simulink model "Target_Control_System"  (R2021b)
settings: Solver=FixedStepDiscrete  StartTime=0.0  StopTime=5  RelTol=1e-3
PreLoadFcn:
  | RTWConfigurationCB('preloadfcn', bdroot);
PostLoadFcn:
  | load('configuration/data_struct.mat');
  | load('configuration/fluxMaps_propMotor.mat');
  | load('configuration/parameterInit_PROP.mat');
  | load('configuration/parameterInit_PUMP.mat');
  | load('configuration/parameterInit_PITCH.mat');
  | load('configuration/parameterInit_TILT.mat');
  | %load('configuration/base_workspace_signal_definition.mat');
  | %load('resolvedatastores_to_baseworkspace_for_faster_simulation.mat');
model workspace (MAT data in the model file):
  SIMULATION_OPTIONS : Simulink.Parameter (value not decoded)
  TARGET_CODE_GEN : Simulink.Parameter (value not decoded)
  TCS_SAMPLE_FREQ_HZ : Simulink.Parameter (value not decoded)
symbols that are objects in the model workspace (value not decoded): TARGET_CODE_GEN, TCS_SAMPLE_FREQ_HZ
undefined symbols (not defined in the file): A_DQ_REF_LPF_INIT__PITCH, A_DQ_REF_LPF_INIT__PROP, A_DQ_REF_LPF_INIT__PUMP, A_DQ_REF_LPF_INIT__TILT, A_OBSERVER_CONFIDENCE_INIT__PITCH, A_OBSERVER_CONFIDENCE_INIT__PROP, A_OBSERVER_CONFIDENCE_INIT__PUMP, A_OBSERVER_CONFIDENCE_INIT__TILT, ACTUATOR_MAX_ANGLE_TRIP__PITCH, ACTUATOR_MIN_ANGLE_TRIP__PITCH, ACTUATOR_POS_SENSOR_INV_DIRECTION__PITCH, ACTUATOR_POS_SENSOR_INV_DIRECTION__TILT, ACTUATOR_POS_SENSOR_OFFSET__PITCH, ACTUATOR_POS_SENSOR_OFFSET__TILT, ADC_scaler1_baseaddr_TILT, ADC_SCALER_FLOAT_TO_FIXPOINT_EXPANSION, ANGLE_ELEC_FROM_SENSOR_OFFSET_INIT__PITCH, ANGLE_ELEC_FROM_SENSOR_OFFSET_INIT__PROP, ANGLE_ELEC_FROM_SENSOR_OFFSET_INIT__PUMP, ANGLE_ELEC_FROM_SENSOR_OFFSET_INIT__TILT, AUTO_CLEAR_FAULTS_ENABLED__PITCH, AUTO_CLEAR_FAULTS_ENABLED__PROP, AUTO_CLEAR_FAULTS_ENABLED__PUMP, AUTO_CLEAR_FAULTS_ENABLED__TILT, AUTO_CLEAR_FAULTS_WAIT_TICKS__PITCH, AUTO_CLEAR_FAULTS_WAIT_TICKS__PROP, AUTO_CLEAR_FAULTS_WAIT_TICKS__PUMP, AUTO_CLEAR_FAULTS_WAIT_TICKS__TILT, AUTO_I_ZERO_IDLE_TICKS__PITCH, AUTO_I_ZERO_IDLE_TICKS__PROP, AUTO_I_ZERO_IDLE_TICKS__PUMP, AUTO_I_ZERO_IDLE_TICKS__TILT, AUTO_I_ZERO_OFFSET_IDC_THRESHOLD__PITCH, AUTO_I_ZERO_OFFSET_IDC_THRESHOLD__PROP, AUTO_I_ZERO_OFFSET_IDC_THRESHOLD__PUMP, AUTO_I_ZERO_OFFSET_IDC_THRESHOLD__TILT, AUTO_I_ZERO_OFFSET_IPH_THRESHOLD__PITCH, AUTO_I_ZERO_OFFSET_IPH_THRESHOLD__PROP, AUTO_I_ZERO_OFFSET_IPH_THRESHOLD__PUMP, AUTO_I_ZERO_OFFSET_IPH_THRESHOLD__TILT, AUTO_SENSORLESS_SWITCHOVER_DISABLE_OMEGA, AUTO_SENSORLESS_SWITCHOVER_ENABLE_OMEGA, AUTO_SENSORLESS_SWITCHOVER_MIN_CONFIDENCE, AUXILIARY_PROTECTION_UNIT_BASEADDR__TILT, blanking_max_error_omega_INIT_PITCH, blanking_max_error_omega_INIT_TILT, blanking_max_error_position_INIT_PITCH, blanking_max_error_position_INIT_TILT, BRUTE_START_I_Q_REF_RAMP_SPEED__PITCH, BRUTE_START_I_Q_REF_RAMP_SPEED__PROP, BRUTE_START_I_Q_REF_RAMP_SPEED__PUMP, BRUTE_START_I_Q_REF_RAMP_SPEED__TILT, CONTROL_LOOP_DT_INIT__PITCH, CONTROL_LOOP_DT_INIT__PROP, CONTROL_LOOP_DT_INIT__PUMP, CONTROL_LOOP_DT_INIT__TILT, CORRECTION_FILTER_SCALE__PITCH, CORRECTION_FILTER_SCALE__PROP, CORRECTION_FILTER_SCALE__PUMP, CORRECTION_FILTER_SCALE__TILT ... (+458)
libraries: simulink x178, Reusables_Lib x24
(part 42 of 47)

== system Target_Control_System/Target_Control_System/MainLoop/tiltMotor_mainLoop/mainTask_tilt/motorTaskMainFastStep(&oTilt)/Mechanical System - Tilt/processSensors(&oPitch)/Input (motor) side sensor/PosSensorProcess_altImplementations/If Action Subsystem1 ==
  Action Port : ActionPort
  Add6 : Sum
  Constant10 : Constant  Value=-1.5*pi
  Constant11 : Constant  Value=2.0*pi
  Constant9 : Constant  Value=2.0*pi
  Data Store Read20 : DataStoreRead  DataStoreName=oTilt  DataStoreElements=oTilt.oMot_.oState_.oPosSensor_.fAngleElecFromSensor_  IndexOptions=Index vector (dialog)  Indices=1  OutputSizes=1
  Data Store Read21 : DataStoreRead  DataStoreName=oTilt  DataStoreElements=oTilt.oMot_.oState_.oPosSensor_.fAngleElecFromSensorPrevious_  IndexOptions=Index vector (dialog)  Indices=1  OutputSizes=1
  Data Store Read22 : DataStoreRead  DataStoreName=oTilt  DataStoreElements=oTilt.oMot_.oParam_.fIntControlLoopDt_  IndexOptions=Index vector (dialog)  Indices=1  OutputSizes=1
  Data Store Read23 : DataStoreRead  DataStoreName=oTilt  DataStoreElements=oTilt.oMot_.oState_.oPosSensor_.oInputSensorSpeedFilter_.afConstantsA_.h0  IndexOptions=Index vector (dialog)  Indices=1  OutputSizes=1
  Data Store Read24 : DataStoreRead  DataStoreName=oTilt  DataStoreElements=oTilt.oMot_.oState_.oPosSensor_.oInputSensorSpeedFilter_.afConstantsA_.h1  IndexOptions=Index vector (dialog)  Indices=1  OutputSizes=1
  Data Store Read25 : DataStoreRead  DataStoreName=oTilt  DataStoreElements=oTilt.oMot_.oState_.oPosSensor_.oInputSensorSpeedFilter_.afConstantsA_.h2  IndexOptions=Index vector (dialog)  Indices=1  OutputSizes=1
  Data Store Read26 : DataStoreRead  DataStoreName=oTilt  DataStoreElements=oTilt.oMot_.oState_.oPosSensor_.oInputSensorSpeedFilter_.afConstantsB_.h0  IndexOptions=Index vector (dialog)  Indices=1  OutputSizes=1
  Data Store Read27 : DataStoreRead  DataStoreName=oTilt  DataStoreElements=oTilt.oMot_.oState_.oPosSensor_.oInputSensorSpeedFilter_.afConstantsB_.h1  IndexOptions=Index vector (dialog)  Indices=1  OutputSizes=1
  Data Store Read28 : DataStoreRead  DataStoreName=oTilt  DataStoreElements=oTilt.oMot_.oState_.oPosSensor_.oInputSensorSpeedFilter_.afConstantsB_.h2  IndexOptions=Index vector (dialog)  Indices=1  OutputSizes=1
  Data Store Read29 : DataStoreRead  DataStoreName=oTilt  DataStoreElements=oTilt.oMot_.oState_.oPosSensor_.oInputSensorSpeedFilter_.afPreviousInputs_.h0  IndexOptions=Index vector (dialog)  Indices=1  OutputSizes=1
  Data Store Read30 : DataStoreRead  DataStoreName=oTilt  DataStoreElements=oTilt.oMot_.oState_.oPosSensor_.oInputSensorSpeedFilter_.afPreviousInputs_.h1  IndexOptions=Index vector (dialog)  Indices=1  OutputSizes=1
  Data Store Read31 : DataStoreRead  DataStoreName=oTilt  DataStoreElements=oTilt.oMot_.oState_.oPosSensor_.oInputSensorSpeedFilter_.afPreviousOutputs_.h0  IndexOptions=Index vector (dialog)  Indices=1  OutputSizes=1
  Data Store Read32 : DataStoreRead  DataStoreName=oTilt  DataStoreElements=oTilt.oMot_.oState_.oPosSensor_.oInputSensorSpeedFilter_.afPreviousOutputs_.h1  IndexOptions=Index vector (dialog)  Indices=1  OutputSizes=1
  Data Store Write5 : DataStoreWrite  DataStoreName=oTilt  DataStoreElements=oTilt.oMot_.oState_.oPosSensor_.oInputSensorSpeedFilter_.fFilterOutput_  IndexOptions=Index vector (dialog)  Indices=1  OutputSizes=1
  Data Store Write6 : DataStoreWrite  DataStoreName=oTilt  DataStoreElements=oTilt.oMot_.oState_.oPosSensor_.oInputSensorSpeedFilter_.afPreviousOutputs_.h0  IndexOptions=Index vector (dialog)  Indices=1  OutputSizes=1
  Data Store Write7 : DataStoreWrite  DataStoreName=oTilt  DataStoreElements=oTilt.oMot_.oState_.oPosSensor_.oInputSensorSpeedFilter_.afPreviousOutputs_.h1  IndexOptions=Index vector (dialog)  Indices=1  OutputSizes=1
  Data Store Write8 : DataStoreWrite  DataStoreName=oTilt  DataStoreElements=oTilt.oMot_.oState_.oPosSensor_.oInputSensorSpeedFilter_.afPreviousInputs_.h0  IndexOptions=Index vector (dialog)  Indices=1  OutputSizes=1
  Data Store Write9 : DataStoreWrite  DataStoreName=oTilt  DataStoreElements=oTilt.oMot_.oState_.oPosSensor_.oInputSensorSpeedFilter_.afPreviousInputs_.h1  IndexOptions=Index vector (dialog)  Indices=1  OutputSizes=1
  Data Type Conversion : DataTypeConversion  OutDataTypeStr=single
  Data Type Conversion1 : DataTypeConversion  OutDataTypeStr=single
  Data Type Conversion2 : DataTypeConversion  OutDataTypeStr=single
  Divide : Product  Inputs=*/
  Less Than : RelationalOperator  Operator=<  OutDataTypeStr=boolean  RndMeth=Simplest
  Subtract6 : Sum  Inputs=+-
  Subtract7 : Sum  Inputs=+-
  Switch6 : Switch  Criteria=u2 > Threshold  Threshold=1.5*pi
  Switch7 : Switch  Criteria=u2 > Threshold
  softwareIirFilterStep() : Subsystem
  fFilterOutput : Outport
  wires:
  Data Type Conversion2/1 -> Data Store Write5/1, fFilterOutput/1
  Data Type Conversion1/1 -> Data Store Write6/1
  Data Type Conversion/1 -> Data Store Write8/1
  Switch7/1 -> Divide/1
  Data Store Read28/1 -> softwareIirFilterStep()/4(afConstantsB2)
  softwareIirFilterStep()/2(*afPreviousInputs0) -> Data Type Conversion/1
  Data Store Read21/1 -> Subtract6/2
  Subtract6/1 -> Switch6/2, Subtract7/1, Switch6/3
  Data Store Read24/1 -> softwareIirFilterStep()/6(afConstantsA1)
  Data Store Read29/1 -> softwareIirFilterStep()/8(afPreviousInputs0)
  Add6/1 -> Switch7/1
  softwareIirFilterStep()/4(*afPreviousOutputs0) -> Data Type Conversion1/1
  Data Store Read22/1 -> Divide/2
  Divide/1 -> softwareIirFilterStep()/1(newInput)
  Data Store Read20/1 -> Subtract6/1
  softwareIirFilterStep()/3(*afPreviousOutputs1) -> Data Store Write7/1
  Constant9/1 -> Subtract7/2
  Data Store Read26/1 -> softwareIirFilterStep()/2(afConstantsB0)
  Switch6/1 -> Less Than/1, Switch7/3, Add6/2
  Data Store Read32/1 -> softwareIirFilterStep()/11(afPreviousOutputs1)
  Data Store Read30/1 -> softwareIirFilterStep()/9(afPreviousInputs1)
  softwareIirFilterStep()/1(*afPreviousInputs1) -> Data Store Write9/1
  Subtract7/1 -> Switch6/1
  Data Store Read25/1 -> softwareIirFilterStep()/7(afConstantsA2)
  Data Store Read27/1 -> softwareIirFilterStep()/3(afConstantsB1)
  Data Store Read23/1 -> softwareIirFilterStep()/5(afConstantsA0)
  Less Than/1 -> Switch7/2
  Constant10/1 -> Less Than/2
  Data Store Read31/1 -> softwareIirFilterStep()/10(afPreviousOutputs0)
  Constant11/1 -> Add6/1
  softwareIirFilterStep()/5(fFilterOutput) -> Data Type Conversion2/1

== system Target_Control_System/Target_Control_System/MainLoop/tiltMotor_mainLoop/mainTask_tilt/motorTaskMainFastStep(&oTilt)/Mechanical System - Tilt/processSensors(&oPitch)/Input (motor) side sensor/PosSensorProcess_altImplementations/Triggered Subsystem ==
  In1 : Inport
  Trigger : TriggerPort  VariantControl=Variant
  Out1 : Outport
  wires:
  In1/1 -> Out1/1

== system Target_Control_System/Target_Control_System/MainLoop/tiltMotor_mainLoop/mainTask_tilt/motorTaskMainFastStep(&oTilt)/Mechanical System - Tilt/processSensors(&oPitch)/Input (motor) side sensor/PosSensorProcess_altImplementations/Triggered Subsystem1 ==
  In1 : Inport
  Trigger : TriggerPort  VariantControl=Variant
  Out1 : Outport
  wires:
  In1/1 -> Out1/1

== system Target_Control_System/Target_Control_System/MainLoop/tiltMotor_mainLoop/mainTask_tilt/motorTaskMainFastStep(&oTilt)/Mechanical System - Tilt/processSensors(&oPitch)/Input (motor) side sensor/PosSensorProcess_altImplementations/While Iterator Subsystem ==
  In1 : Inport
  IC : Inport  Port=2
  Constant : Constant  OutDataTypeStr=single
  Constant4 : Constant  Value=2*pi  OutDataTypeStr=single
  Data Store Read1 : DataStoreRead  DataStoreName=oTilt  DataStoreElements=oTilt.oMot_.oState_.oPosSensor_.iAngleMechToElecWrappings_  IndexOptions=Index vector (dialog)  Indices=1  OutputSizes=1
  Data Store Read13 : DataStoreRead  DataStoreName=oTilt  DataStoreElements=oTilt.oMot_.oState_.oPosSensor_.fAngleElecFromSensor_  IndexOptions=Index vector (dialog)  Indices=1  OutputSizes=1
  Data Store Write1 : DataStoreWrite  DataStoreName=oTilt  DataStoreElements=oTilt.oMot_.oState_.oPosSensor_.fAngleElecFromSensor_  IndexOptions=Index vector (dialog)  Indices=1  OutputSizes=1
  Data Store Write2 : DataStoreWrite  DataStoreName=oTilt  DataStoreElements=oTilt.oMot_.oState_.oPosSensor_.fAngleElecFromSensor_  IndexOptions=Index vector (dialog)  Indices=1  OutputSizes=1
  Subtract : Sum  Inputs=+-  OutDataTypeStr=single
  Subtract1 : Sum  OutDataTypeStr=single
  While Iterator : WhileIterator  MaxIters=100  ResetStates=reset  ShowIterationPort=on
  Out1 : Outport
  wires:
  Subtract1/1 -> Data Store Write1/1
  While Iterator/1 -> Out1/1
  Constant/1 -> Subtract1/2
  Data Store Read1/1 -> Subtract1/1
  Constant4/1 -> Subtract/2
  Subtract/1 -> Data Store Write2/1
  In1/1 -> While Iterator/1
  Data Store Read13/1 -> Subtract/1
  IC/1 -> While Iterator/2

== system Target_Control_System/Target_Control_System/MainLoop/tiltMotor_mainLoop/mainTask_tilt/motorTaskMainFastStep(&oTilt)/Mechanical System - Tilt/processSensors(&oPitch)/Input (motor) side sensor/PosSensorProcess_altImplementations/While Iterator Subsystem1 ==
  In1 : Inport
  IC : Inport  Port=2
  Constant : Constant  OutDataTypeStr=single
  Constant4 : Constant  Value=2*pi  OutDataTypeStr=single
  Data Store Read1 : DataStoreRead  DataStoreName=oTilt  DataStoreElements=oTilt.oMot_.oState_.oPosSensor_.iAngleMechToElecWrappings_  IndexOptions=Index vector (dialog)  Indices=1  OutputSizes=1
  Data Store Read13 : DataStoreRead  DataStoreName=oTilt  DataStoreElements=oTilt.oMot_.oState_.oPosSensor_.fAngleElecFromSensor_  IndexOptions=Index vector (dialog)  Indices=1  OutputSizes=1
  Data Store Write1 : DataStoreWrite  DataStoreName=oTilt  DataStoreElements=oTilt.oMot_.oState_.oPosSensor_.fAngleElecFromSensor_  IndexOptions=Index vector (dialog)  Indices=1  OutputSizes=1
  Data Store Write2 : DataStoreWrite  DataStoreName=oTilt  DataStoreElements=oTilt.oMot_.oState_.oPosSensor_.fAngleElecFromSensor_  IndexOptions=Index vector (dialog)  Indices=1  OutputSizes=1
  Subtract : Sum  OutDataTypeStr=single
  Subtract1 : Sum  Inputs=+-  OutDataTypeStr=single
  While Iterator : WhileIterator  MaxIters=100  ResetStates=reset  ShowIterationPort=on
  Out1 : Outport
  wires:
  While Iterator/1 -> Out1/1
  Constant/1 -> Subtract1/2
  Subtract1/1 -> Data Store Write1/1
  Data Store Read1/1 -> Subtract1/1
  Constant4/1 -> Subtract/2
  Subtract/1 -> Data Store Write2/1
  In1/1 -> While Iterator/1
  Data Store Read13/1 -> Subtract/1
  IC/1 -> While Iterator/2

== system Target_Control_System/Target_Control_System/MainLoop/tiltMotor_mainLoop/mainTask_tilt/motorTaskMainFastStep(&oTilt)/Mechanical System - Tilt/processSensors(&oPitch)/Input (motor) side sensor/updateGbxOutput/updateAngles ==
  fCurrentOutputAngle : Inport
  fNewInputAngle : Inport  Port=2
  Data Store Write : DataStoreWrite  DataStoreName=oTilt  DataStoreElements=oTilt.oMot_.oState_.oPosSensor_.oGbx_.fCurrentOutputAngle_  IndexOptions=Index vector (dialog)  Indices=1  OutputSizes=1
  Data Store Write1 : DataStoreWrite  DataStoreName=oTilt  DataStoreElements=oTilt.oMot_.oState_.oPosSensor_.oGbx_.fPreviousInputAngle_  IndexOptions=Index vector (dialog)  Indices=1  OutputSizes=1
  wires:
  fNewInputAngle/1 -> Data Store Write1/1
  fCurrentOutputAngle/1 -> Data Store Write/1

== system Target_Control_System/Target_Control_System/MainLoop/tiltMotor_mainLoop/mainTask_tilt/motorTaskMainFastStep(&oTilt)/Software Overcurrent Protection - Tilt/checkForHwOvercurrents(&oTilt)/gateDriverStatus/IncludeCustomCode/System Update ==

== system Target_Control_System/Target_Control_System/MainLoop/pitchMotor_mainLoop/Decimation gate for 200 Hz Pitch/Function-Call Subsystem/Position control checks/Position control mode/checkSensorLimits(&oPitch)/Read sensor flags/nonresolverSensorCodes/ModelSource ==
  note: 1) Add Subsystem or Model blocks as valid variant choices.
      | 2) You cannot connect blocks at this level. At simulation, connectivity is automatically
      | determined, based on the active variant and port name matching.
  DoNotIncludeCustomCode : Subsystem  TreatAsAtomicUnit=on  VariantControl=TARGET_CODE_GEN == 0
  IncludeCustomCode : Subsystem  TreatAsAtomicUnit=on  VariantControl=(default)

== system Target_Control_System/Target_Control_System/MainLoop/pitchMotor_mainLoop/Decimation gate for 200 Hz Pitch/Function-Call Subsystem/Position control checks/Position control mode/checkSensorLimits(&oPitch)/Read sensor flags/resolverSensorCodes/ModelSource ==
  note: 1) Add Subsystem or Model blocks as valid variant choices.
      | 2) You cannot connect blocks at this level. At simulation, connectivity is automatically
      | determined, based on the active variant and port name matching.
  DoNotIncludeCustomCode : Subsystem  TreatAsAtomicUnit=on  VariantControl=TARGET_CODE_GEN == 0
  IncludeCustomCode : Subsystem  TreatAsAtomicUnit=on  VariantControl=(default)

== system Target_Control_System/Target_Control_System/MainLoop/pitchMotor_mainLoop/mainTask_pitch/motorTaskMainFastStep()/Mechanical System - Pitch/processSensors(&oPitch)/Input (motor) side sensor/Compute Speed From Sensor/softwareIirFilterStep()/prepare for next round ==
  fOutput_in : Inport
  fNewInput : Inport  Port=2
  Data Store Read : DataStoreRead  DataStoreName=oPitch  DataStoreElements=oPitch.oMot_.oState_.oPosSensor_.oInputSensorSpeedFilter_.afPreviousInputs_.h0  IndexOptions=Index vector (dialog)  Indices=1  OutputSizes=1
  Data Store Read6 : DataStoreRead  DataStoreName=oPitch  DataStoreElements=oPitch.oMot_.oState_.oPosSensor_.oInputSensorSpeedFilter_.afPreviousOutputs_.h0  IndexOptions=Index vector (dialog)  Indices=1  OutputSizes=1
  Data Store Write : DataStoreWrite  DataStoreName=oPitch  DataStoreElements=oPitch.oMot_.oState_.oPosSensor_.oInputSensorSpeedFilter_.afPreviousInputs_.h1  IndexOptions=Index vector (dialog)  Indices=1  OutputSizes=1
  Data Store Write1 : DataStoreWrite  DataStoreName=oPitch  DataStoreElements=oPitch.oMot_.oState_.oPosSensor_.oInputSensorSpeedFilter_.afPreviousInputs_.h0  IndexOptions=Index vector (dialog)  Indices=1  OutputSizes=1
  Data Store Write2 : DataStoreWrite  DataStoreName=oPitch  DataStoreElements=oPitch.oMot_.oState_.oPosSensor_.oInputSensorSpeedFilter_.afPreviousOutputs_.h1  IndexOptions=Index vector (dialog)  Indices=1  OutputSizes=1
  Data Store Write3 : DataStoreWrite  DataStoreName=oPitch  DataStoreElements=oPitch.oMot_.oState_.oPosSensor_.oInputSensorSpeedFilter_.afPreviousOutputs_.h0  IndexOptions=Index vector (dialog)  Indices=1  OutputSizes=1
  fOutput : Outport
  wires:
  fOutput_in/1 -> Data Store Write3/1, fOutput/1
  Data Store Read6/1 -> Data Store Write2/1
  fNewInput/1 -> Data Store Write1/1
  Data Store Read/1 -> Data Store Write/1

== system Target_Control_System/Target_Control_System/MainLoop/tiltMotor_mainLoop/Decimation gate for 200 Hz Tilt/motorTaskMainDecimationAStep(&oTilt)/Position control checks/Position control mode/checkSensorLimits(&oTilt)/Read sensor flags/nonresolverSensorCodes/ModelSource ==
  note: 1) Add Subsystem or Model blocks as valid variant choices.
      | 2) You cannot connect blocks at this level. At simulation, connectivity is automatically
      | determined, based on the active variant and port name matching.
  DoNotIncludeCustomCode : Subsystem  TreatAsAtomicUnit=on  VariantControl=TARGET_CODE_GEN == 0
  IncludeCustomCode : Subsystem  TreatAsAtomicUnit=on  VariantControl=(default)

== system Target_Control_System/Target_Control_System/MainLoop/tiltMotor_mainLoop/Decimation gate for 200 Hz Tilt/motorTaskMainDecimationAStep(&oTilt)/Position control checks/Position control mode/checkSensorLimits(&oTilt)/Read sensor flags/resolverSensorCodes/ModelSource ==
  note: 1) Add Subsystem or Model blocks as valid variant choices.
      | 2) You cannot connect blocks at this level. At simulation, connectivity is automatically
      | determined, based on the active variant and port name matching.
  DoNotIncludeCustomCode : Subsystem  TreatAsAtomicUnit=on  VariantControl=TARGET_CODE_GEN == 0
  IncludeCustomCode : Subsystem  TreatAsAtomicUnit=on  VariantControl=(default)

== system Target_Control_System/Target_Control_System/MainLoop/tiltMotor_mainLoop/mainTask_tilt/motorTaskMainFastStep(&oTilt)/Mechanical System - Tilt/processSensors(&oPitch)/Input (motor) side sensor/Compute Speed From Sensor/softwareIirFilterStep()1/prepare for next round ==
  fOutput_in : Inport
  fNewInput : Inport  Port=2
  Data Store Read : DataStoreRead  DataStoreName=oTilt  DataStoreElements=oTilt.oMot_.oState_.oPosSensor_.oInputSensorSpeedFilter_.afPreviousInputs_.h0  IndexOptions=Index vector (dialog)  Indices=1  OutputSizes=1
  Data Store Read6 : DataStoreRead  DataStoreName=oTilt  DataStoreElements=oTilt.oMot_.oState_.oPosSensor_.oInputSensorSpeedFilter_.afPreviousOutputs_.h0  IndexOptions=Index vector (dialog)  Indices=1  OutputSizes=1
  Data Store Write : DataStoreWrite  DataStoreName=oTilt  DataStoreElements=oTilt.oMot_.oState_.oPosSensor_.oInputSensorSpeedFilter_.afPreviousInputs_.h1  IndexOptions=Index vector (dialog)  Indices=1  OutputSizes=1
  Data Store Write1 : DataStoreWrite  DataStoreName=oTilt  DataStoreElements=oTilt.oMot_.oState_.oPosSensor_.oInputSensorSpeedFilter_.afPreviousInputs_.h0  IndexOptions=Index vector (dialog)  Indices=1  OutputSizes=1
  Data Store Write2 : DataStoreWrite  DataStoreName=oTilt  DataStoreElements=oTilt.oMot_.oState_.oPosSensor_.oInputSensorSpeedFilter_.afPreviousOutputs_.h1  IndexOptions=Index vector (dialog)  Indices=1  OutputSizes=1
  Data Store Write3 : DataStoreWrite  DataStoreName=oTilt  DataStoreElements=oTilt.oMot_.oState_.oPosSensor_.oInputSensorSpeedFilter_.afPreviousOutputs_.h0  IndexOptions=Index vector (dialog)  Indices=1  OutputSizes=1
  fOutput : Outport
  wires:
  fOutput_in/1 -> Data Store Write3/1, fOutput/1
  Data Store Read6/1 -> Data Store Write2/1
  fNewInput/1 -> Data Store Write1/1
  Data Store Read/1 -> Data Store Write/1

== system Target_Control_System/Target_Control_System/MainLoop/tiltMotor_mainLoop/mainTask_tilt/motorTaskMainFastStep(&oTilt)/Mechanical System - Tilt/processSensors(&oPitch)/Input (motor) side sensor/PosSensorProcess_altImplementations/If Action Subsystem1/softwareIirFilterStep() ==
  newInput : Inport
  afConstantsB0 : Inport  Port=2
  afConstantsB1 : Inport  Port=3
  afConstantsB2 : Inport  Port=4
  afConstantsA0 : Inport  Port=5
  afConstantsA1 : Inport  Port=6
  afConstantsA2 : Inport  Port=7
  afPreviousInputs0 : Inport  Port=8
  afPreviousInputs1 : Inport  Port=9
  afPreviousOutputs0 : Inport  Port=10
  afPreviousOutputs1 : Inport  Port=11
  Add : Sum  Inputs=+++--
  Constant : Constant  Value=0  OutDataTypeStr=single
  Constant1 : Constant  Value=0  OutDataTypeStr=single
  Divide{,1..5} (6 alike) : Product  Inputs=**
  IsInf : RelationalOperator  Operator=isInf  OutDataTypeStr=boolean  RndMeth=Simplest
  IsInf1 : RelationalOperator  Operator=isInf  OutDataTypeStr=boolean  RndMeth=Simplest
  IsNaN : RelationalOperator  Operator=isNaN  OutDataTypeStr=boolean  RndMeth=Simplest
  IsNaN1 : RelationalOperator  Operator=isNaN  OutDataTypeStr=boolean  RndMeth=Simplest
  Switch{,1..3} (4 alike) : Switch  Criteria=u2 > Threshold
  *afPreviousInputs1 : Outport
  *afPreviousInputs0 : Outport  Port=2
  *afPreviousOutputs1 : Outport  Port=3
  *afPreviousOutputs0 : Outport  Port=4
  fFilterOutput : Outport  Port=5
  wires:
  Switch3/1 -> Divide5/1, *afPreviousOutputs0/1
  IsInf1/1 -> Switch3/2
  IsNaN1/1 -> Switch2/2
  Constant1/1 -> Switch2/1, Switch3/1
  Switch2/1 -> IsInf1/1, Switch3/3
  Add/1 -> IsNaN1/1, Switch2/3  "fOutput"
  Switch1/1 -> Divide/1, *afPreviousInputs0/1
  Switch/1 -> IsInf/1, Switch1/3
  IsInf/1 -> Switch1/2
  Constant/1 -> Switch/1, Switch1/1
  IsNaN/1 -> Switch/2
  Divide5/1 -> fFilterOutput/1
  afConstantsA0/1 -> Divide5/2
  afPreviousOutputs1/1 -> Divide4/1
  afConstantsA2/1 -> Divide4/2
  afPreviousOutputs0/1 -> Divide3/1, *afPreviousOutputs1/1
  afConstantsA1/1 -> Divide3/2
  afPreviousInputs1/1 -> Divide2/1
  afConstantsB2/1 -> Divide2/2
  Divide4/1 -> Add/5
  Divide3/1 -> Add/4
  Divide/1 -> Add/1
  Divide1/1 -> Add/2
  Divide2/1 -> Add/3
  afPreviousInputs0/1 -> Divide1/1, *afPreviousInputs1/1
  afConstantsB1/1 -> Divide1/2
  newInput/1 -> IsNaN/1, Switch/3
  afConstantsB0/1 -> Divide/2

== system Target_Control_System/Target_Control_System/MainLoop/pitchMotor_mainLoop/Decimation gate for 200 Hz Pitch/Function-Call Subsystem/Position control checks/Position control mode/checkSensorLimits(&oPitch)/Read sensor flags/nonresolverSensorCodes/ModelSource/DoNotIncludeCustomCode ==
  Constant : Constant  Value=0  OutDataTypeStr=uint32  SampleTime=-1
  Constant1 : Constant  OutDataTypeStr=uint32  SampleTime=-1
  Data Store Write : DataStoreWrite  DataStoreName=mdl_pitch_uiInputSensorFlags  IndexOptions=Index vector (dialog)  Indices=1  OutputSizes=1
  Data Store Write1 : DataStoreWrite  DataStoreName=mdl_pitch_uiOutputSensorFlags  IndexOptions=Index vector (dialog)  Indices=1  OutputSizes=1
  wires:
  Constant1/1 -> Data Store Write1/1
  Constant/1 -> Data Store Write/1

== system Target_Control_System/Target_Control_System/MainLoop/pitchMotor_mainLoop/Decimation gate for 200 Hz Pitch/Function-Call Subsystem/Position control checks/Position control mode/checkSensorLimits(&oPitch)/Read sensor flags/nonresolverSensorCodes/ModelSource/IncludeCustomCode ==
  System Update : Subsystem  mask(System Update){ShowInLibBrowser=0}
      mask prompts: ShowInLibBrowser "Simulink:masks:CustCodeMaskParam1_MP"
      settings: CopyFcn=cccopyfcn(gcb)  OpenFcn=ccopenfcn('System Update Function')
      mask Help: eval('feval(''rtwprivate'',''rtwhelpview'',''rtw_sys_update_block'')');
      mask DialogControl ShowInLibBrowser Prompt: Mask Parameter 1:
      mask Display: disp('System\nUpdate');

== system Target_Control_System/Target_Control_System/MainLoop/pitchMotor_mainLoop/Decimation gate for 200 Hz Pitch/Function-Call Subsystem/Position control checks/Position control mode/checkSensorLimits(&oPitch)/Read sensor flags/resolverSensorCodes/ModelSource/DoNotIncludeCustomCode ==
  Constant : Constant  Value=0  OutDataTypeStr=uint32  SampleTime=-1
  Constant1 : Constant  OutDataTypeStr=uint32  SampleTime=-1
  Data Store Write : DataStoreWrite  DataStoreName=mdl_pitch_uiInputSensorFlags  IndexOptions=Index vector (dialog)  Indices=1  OutputSizes=1
  Data Store Write1 : DataStoreWrite  DataStoreName=mdl_pitch_uiOutputSensorFlags  IndexOptions=Index vector (dialog)  Indices=1  OutputSizes=1
  wires:
  Constant1/1 -> Data Store Write1/1
  Constant/1 -> Data Store Write/1

== system Target_Control_System/Target_Control_System/MainLoop/pitchMotor_mainLoop/Decimation gate for 200 Hz Pitch/Function-Call Subsystem/Position control checks/Position control mode/checkSensorLimits(&oPitch)/Read sensor flags/resolverSensorCodes/ModelSource/IncludeCustomCode ==
  System Update : Subsystem  mask(System Update){ShowInLibBrowser=0}
      mask prompts: ShowInLibBrowser "Simulink:masks:CustCodeMaskParam1_MP"
      settings: CopyFcn=cccopyfcn(gcb)  OpenFcn=ccopenfcn('System Update Function')
      mask Help: eval('feval(''rtwprivate'',''rtwhelpview'',''rtw_sys_update_block'')');
      mask DialogControl ShowInLibBrowser Prompt: Mask Parameter 1:
      mask Display: disp('System\nUpdate');

== system Target_Control_System/Target_Control_System/MainLoop/tiltMotor_mainLoop/Decimation gate for 200 Hz Tilt/motorTaskMainDecimationAStep(&oTilt)/Position control checks/Position control mode/checkSensorLimits(&oTilt)/Read sensor flags/nonresolverSensorCodes/ModelSource/DoNotIncludeCustomCode ==

== system Target_Control_System/Target_Control_System/MainLoop/tiltMotor_mainLoop/Decimation gate for 200 Hz Tilt/motorTaskMainDecimationAStep(&oTilt)/Position control checks/Position control mode/checkSensorLimits(&oTilt)/Read sensor flags/nonresolverSensorCodes/ModelSource/IncludeCustomCode ==
  System Update : Subsystem  mask(System Update){ShowInLibBrowser=0}
      mask prompts: ShowInLibBrowser "Simulink:masks:CustCodeMaskParam1_MP"
      settings: CopyFcn=cccopyfcn(gcb)  OpenFcn=ccopenfcn('System Update Function')
      mask Help: eval('feval(''rtwprivate'',''rtwhelpview'',''rtw_sys_update_block'')');
      mask DialogControl ShowInLibBrowser Prompt: Mask Parameter 1:
      mask Display: disp('System\nUpdate');

== system Target_Control_System/Target_Control_System/MainLoop/tiltMotor_mainLoop/Decimation gate for 200 Hz Tilt/motorTaskMainDecimationAStep(&oTilt)/Position control checks/Position control mode/checkSensorLimits(&oTilt)/Read sensor flags/resolverSensorCodes/ModelSource/DoNotIncludeCustomCode ==

== system Target_Control_System/Target_Control_System/MainLoop/tiltMotor_mainLoop/Decimation gate for 200 Hz Tilt/motorTaskMainDecimationAStep(&oTilt)/Position control checks/Position control mode/checkSensorLimits(&oTilt)/Read sensor flags/resolverSensorCodes/ModelSource/IncludeCustomCode ==
  System Update : Subsystem  mask(System Update){ShowInLibBrowser=0}
      mask prompts: ShowInLibBrowser "Simulink:masks:CustCodeMaskParam1_MP"
      settings: CopyFcn=cccopyfcn(gcb)  OpenFcn=ccopenfcn('System Update Function')
      mask Help: eval('feval(''rtwprivate'',''rtwhelpview'',''rtw_sys_update_block'')');
      mask DialogControl ShowInLibBrowser Prompt: Mask Parameter 1:
      mask Display: disp('System\nUpdate');

== system Target_Control_System/Target_Control_System/MainLoop/pitchMotor_mainLoop/Decimation gate for 200 Hz Pitch/Function-Call Subsystem/Position control checks/Position control mode/checkSensorLimits(&oPitch)/Read sensor flags/nonresolverSensorCodes/ModelSource/IncludeCustomCode/System Update ==

== system Target_Control_System/Target_Control_System/MainLoop/pitchMotor_mainLoop/Decimation gate for 200 Hz Pitch/Function-Call Subsystem/Position control checks/Position control mode/checkSensorLimits(&oPitch)/Read sensor flags/resolverSensorCodes/ModelSource/IncludeCustomCode/System Update ==

== system Target_Control_System/Target_Control_System/MainLoop/tiltMotor_mainLoop/Decimation gate for 200 Hz Tilt/motorTaskMainDecimationAStep(&oTilt)/Position control checks/Position control mode/checkSensorLimits(&oTilt)/Read sensor flags/nonresolverSensorCodes/ModelSource/IncludeCustomCode/System Update ==

== system Target_Control_System/Target_Control_System/MainLoop/tiltMotor_mainLoop/Decimation gate for 200 Hz Tilt/motorTaskMainDecimationAStep(&oTilt)/Position control checks/Position control mode/checkSensorLimits(&oTilt)/Read sensor flags/resolverSensorCodes/ModelSource/IncludeCustomCode/System Update ==

== stateflow chart Target_Control_System/MainLoop/pumpMotor_mainLoop/motorTaskMainFastStep(&oPump)/initiateOffsetNulling(&oPump) ==
  state MainLoopFunctions
    state initiateOffsetNulling [parallel]
      settings: executionOrder=2
      state Disabled
      state Initiate
        entry:
        //We can only do this if idle
        oPump.oIsr_.oState_.fOffsetIntegratorIa_ = 0.0;
        oPump.oIsr_.oState_.fOffsetIntegratorIb_ = 0.0;
        oPump.oIsr_.oState_.fOffsetIntegratorIc_ = 0.0;
        oPump.oIsr_.oState_.fOffsetIntegratorIdc_ = 0.0;
        oPump.oMot_.oState_.uiDriveState_ = 95;
      (default) -> MainLoopFunctions.initiateOffsetNulling.Disabled
      MainLoopFunctions.initiateOffsetNulling.Disabled -> Initiate : [oPump.oMot_.oIn_.uiCurrentOffsetNullingActive_ == 1 ....
          | && (oPump.oMot_.oState_.uiDriveState_ >= 99 ....
          |  || oPump.oMot_.oState_.uiDriveState_ < 102)]
      Initiate -> MainLoopFunctions.initiateOffsetNulling.Disabled : [(oPump.oMot_.oIn_.uiCurrentOffsetNullingActive_ == 0)]
    state initiateVoltageOffsetNulling [parallel]
      settings: executionOrder=1
      state Disabled
      state initiate
        entry:
        // Must do this at 50 % duty
        // Set the offsets to zero:
        fTemp = 0.5F;
        // In the future, there may be reasons to zero the offsets at duties different than 50%.
        // Set the target duty here
        oPump.oMot_.oState_.uiDriveState_ = 245;
        oPump.oMot_.oOut_.uiPwmRequestFromMain_ = 1;
        oPump.oMot_.oOut_.uiPwmDutyTicksFromMainA_ = cast((fTemp * oPump.oMot_.oParam_.fPwmPeriodTicksMainloopFloat_), uint32);
        oPump.oMot_.oOut_.uiPwmDutyTicksFromMainB_ = cast((fTemp * oPump.oMot_.oParam_.fPwmPeriodTicksMainloopFloat_), uint32);
        oPump.oMot_.oOut_.uiPwmDutyTicksFromMainC_ = cast((fTemp * oPump.oMot_.oParam_.fPwmPeriodTicksMainloopFloat_), uint32);
        oPump.oMot_.oOut_.uiEnableGateDrive_ = 0x7;
      (default) -> MainLoopFunctions.initiateVoltageOffsetNulling.Disabled
      MainLoopFunctions.initiateVoltageOffsetNulling.Disabled -> (junction 277) : [oPump.oMot_.oIn_.uiVoltageOffsetNullingActive_ == 1]
      (junction 277) -> MainLoopFunctions.initiateVoltageOffsetNulling.Disabled [order 1] : [oPump.oMot_.oState_.uiDriveState_ < 100 ...
          |  || oPump.oMot_.oState_.uiDriveState_ > 101] ...
          | // Only start if fully idle
      initiate -> MainLoopFunctions.initiateVoltageOffsetNulling.Disabled : [(oPump.oMot_.oIn_.uiVoltageOffsetNullingActive_ == 0)]
      (junction 277) -> initiate [order 2]
  (default) -> MainLoopFunctions
  data: oPump data_store_memory; fTemp local single

== stateflow chart Target_Control_System/MainLoop/propMotor_mainLoop/Decimation gate A for 200 Hz Prop/Current offset nulling/initiateOffsetNulling(&oProp)/Chart ==
  state Start
  state initiateOffsetNulling
    //We can only do this if idle
    entry:
    oProp.oIsr_.oState_.fOffsetIntegratorIa_ = 0.0;
    oProp.oIsr_.oState_.fOffsetIntegratorIb_ = 0.0;
    oProp.oIsr_.oState_.fOffsetIntegratorIc_ = 0.0;
    oProp.oIsr_.oState_.fOffsetIntegratorIdc_ = 0.0;
    oProp.oMot_.oState_.uiDriveState_ = 95;
  (default) -> Start
  initiateOffsetNulling -> Start : [oProp.oMot_.oState_.uiCurrentOffsetNullingPerformed_ == 1]
  Start -> initiateOffsetNulling : [oProp.oMot_.oState_.uiDriveState_ >= 99 && ...
      | oProp.oMot_.oState_.uiDriveState_ < 102]
  data: oProp data_store_memory
